simulink model "seat_sc1"  (R2020a)
settings: Solver=FixedStepDiscrete  StartTime=0.0  StopTime=30  FixedStep=1  RelTol=1e-3
settings Model: Creator=admin  LastModifiedBy=A
settings OptimizationCC: DefaultParameterBehavior=Inlined  EnhancedBackFolding=on  PassReuseOutputArgsAs=Individual arguments  OptimizeBlockOrder=speed  DifferentSizesBufferReuse=on  OptimizationCustomize=off  EfficientTunableParamExpr=on
settings DebuggingCC: ParameterTunabilityLossMsg=error
settings SFSimCC: MATLABDynamicMemAlloc=off  CustomCodeUndefinedFunction=UseInterfaceOnly
settings RTWCC: SystemTargetFile=ert.tlc  TemplateMakefile=ert_default_tmf  GenerateReport=on  IncludeHyperlinkInReport=on  LaunchReport=on  GenerateTraceInfo=on  GenerateTraceReport=on  GenerateTraceReportSl=on  GenerateTraceReportSf=on  GenerateTraceReportEml=on
settings CodeAppCC: ForceParamTrailComments=on  IgnoreCustomStorageClasses=off  OperatorAnnotations=on  SimulinkDataObjDesc=on  SFDataObjDesc=on  InsertBlockDesc=on
settings ERTTargetCC: TargetLangStandard=C99 (ISO)  GenerateSampleERTMain=on  InlinedParameterPlacement=NonHierarchical  ERTCustomFileTemplate=example_file_process.tlc

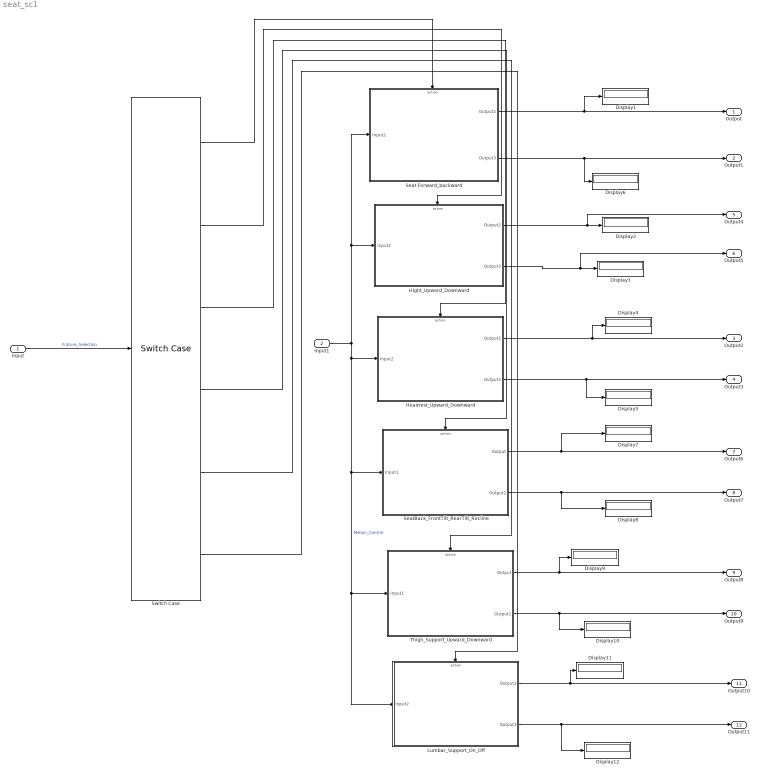
== system seat_sc1 ==
  Input : Inport
  Input1 : Inport  Port=2
  " Seat Forward_backward" : Subsystem  TreatAsAtomicUnit=on
  Display{1..12} (12 alike) : Display
  Headrest_Upward_Downward : Subsystem  TreatAsAtomicUnit=on
  Hight_Upward_Downward : Subsystem  TreatAsAtomicUnit=on
  Lumbar_Support_On_Off : Subsystem  TreatAsAtomicUnit=on
  SeatBack_FrontTilt_RearTilt_Recline : Subsystem  TreatAsAtomicUnit=on
  Switch Case : SwitchCase  CaseConditions={1 2 3 4 5 6}  ShowDefaultCase=off
  Thigh_Support_Upward_Downward : Subsystem  TreatAsAtomicUnit=on
  Output : Outport
  Output1 : Outport  Port=2
  Output2 : Outport  Port=3
  Output3 : Outport  Port=4
  Output4 : Outport  Port=5
  Output5 : Outport  Port=6
  Output6 : Outport  Port=7
  Output7 : Outport  Port=8
  Output8 : Outport  Port=9
  Output9 : Outport  Port=10
  Output10 : Outport  Port=11
  Output11 : Outport  Port=12
  wires:
  Input1/1 -> " Seat Forward_backward"/1(Input2), Hight_Upward_Downward/1(Input2), Lumbar_Support_On_Off/1(Input2), Thigh_Support_Upward_Downward/1(Input1), SeatBack_FrontTilt_RearTilt_Recline/1(Input1), Headrest_Upward_Downward/1(Input2)  "Motion_Control"
  Input/1 -> Switch Case/1  "Frature_Selection"
  Hight_Upward_Downward/1(Output2) -> Output4/1, Display2/1
  Lumbar_Support_On_Off/2(Output3) -> Output11/1, Display12/1
  Switch Case/5 -> Thigh_Support_Upward_Downward/Action
  Thigh_Support_Upward_Downward/1(Output) -> Display9/1, Output8/1
  Thigh_Support_Upward_Downward/2(Output1) -> Output9/1, Display10/1
  Headrest_Upward_Downward/1(Output2) -> Display4/1, Output2/1
  Switch Case/1 -> " Seat Forward_backward"/Action
  SeatBack_FrontTilt_RearTilt_Recline/2(Output1) -> Output7/1, Display8/1
  Switch Case/2 -> Hight_Upward_Downward/Action
  Switch Case/3 -> Headrest_Upward_Downward/Action
  Switch Case/4 -> SeatBack_FrontTilt_RearTilt_Recline/Action
  Lumbar_Support_On_Off/1(Output2) -> Output10/1, Display11/1
  SeatBack_FrontTilt_RearTilt_Recline/1(Output) -> Display7/1, Output6/1
  Switch Case/6 -> Lumbar_Support_On_Off/Action
  " Seat Forward_backward"/1(Output2) -> Display1/1, Output/1
  Headrest_Upward_Downward/2(Output3) -> Output3/1, Display5/1
  Hight_Upward_Downward/2(Output3) -> Output5/1, Display3/1
  " Seat Forward_backward"/2(Output3) -> Display6/1, Output1/1

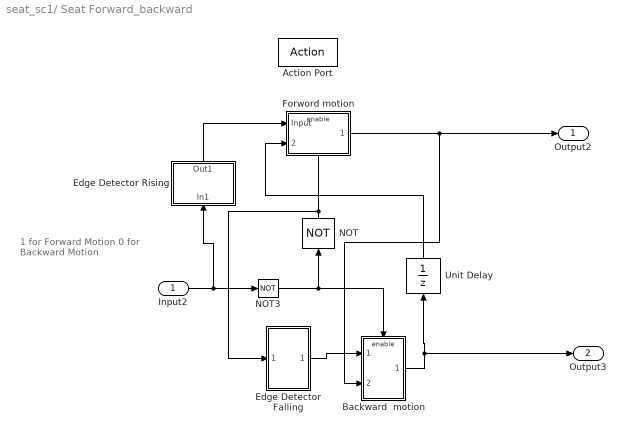
== system seat_sc1/ Seat Forward_backward ==
  note: 1 for Forward Motion
      | 0 for Backward Motion
  Input2 : Inport
  Action Port : ActionPort  ActionPortLabel=case [ 1 ]:
  " Backward  motion" : Subsystem
  Edge Detector Falling : Subsystem  TreatAsAtomicUnit=on
  Edge Detector Rising : Subsystem  TreatAsAtomicUnit=on
  Forword motion : Subsystem
  NOT : Logic  Operator=NOT  IconShape=distinctive  AllPortsSameDT=off  OutDataTypeStr=boolean
  NOT3 : Logic  Operator=NOT  IconShape=distinctive  AllPortsSameDT=off  OutDataTypeStr=boolean
  Unit Delay : UnitDelay  SampleTime=-1  HasFrameUpgradeWarning=on
  Output2 : Outport
  Output3 : Outport  Port=2
  wires:
  " Backward  motion"/1(Output) -> Output3/1, Unit Delay/1
  Edge Detector Falling/1(Out1) -> " Backward  motion"/1(Input)
  Input2/1 -> Edge Detector Rising/1(In1), NOT3/1
  Forword motion/1(Output1) -> " Backward  motion"/2(Input1), Output2/1
  NOT3/1 -> " Backward  motion"/Enable, NOT/1
  NOT/1 -> Forword motion/Enable, Edge Detector Falling/1(In1)
  Edge Detector Rising/1(Out1) -> Forword motion/1(Input)
  Unit Delay/1 -> Forword motion/2(Input1)

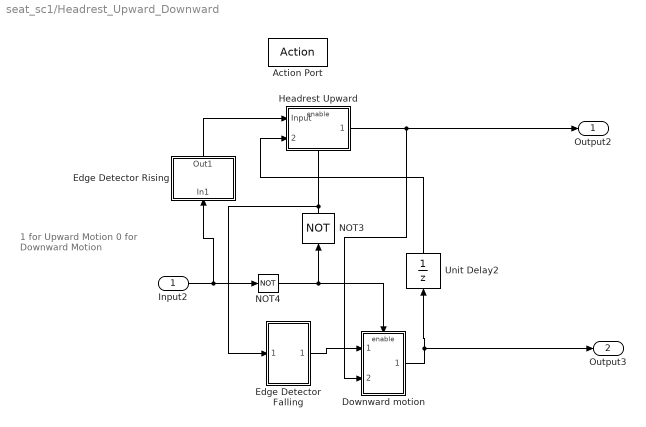
== system seat_sc1/Headrest_Upward_Downward ==
  note: 1 for Upward Motion
      | 0 for Downward Motion
  Input2 : Inport
  Action Port : ActionPort  ActionPortLabel=case [ 3 ]:
  Downward motion : Subsystem
  Edge Detector Falling : Subsystem  TreatAsAtomicUnit=on
  Edge Detector Rising : Subsystem  TreatAsAtomicUnit=on
  Headrest Upward : Subsystem
  NOT3 : Logic  Operator=NOT  IconShape=distinctive  AllPortsSameDT=off  OutDataTypeStr=boolean
  NOT4 : Logic  Operator=NOT  IconShape=distinctive  AllPortsSameDT=off  OutDataTypeStr=boolean
  Unit Delay2 : UnitDelay  SampleTime=-1  HasFrameUpgradeWarning=on
  Output2 : Outport
  Output3 : Outport  Port=2
  wires:
  Unit Delay2/1 -> Headrest Upward/2(Input1)
  Downward motion/1(Output) -> Output3/1, Unit Delay2/1
  Edge Detector Falling/1(Out1) -> Downward motion/1(Input)
  NOT4/1 -> Downward motion/Enable, NOT3/1
  Edge Detector Rising/1(Out1) -> Headrest Upward/1(Input)
  Headrest Upward/1(Output1) -> Downward motion/2(Input1), Output2/1
  NOT3/1 -> Headrest Upward/Enable, Edge Detector Falling/1(In1)
  Input2/1 -> Edge Detector Rising/1(In1), NOT4/1

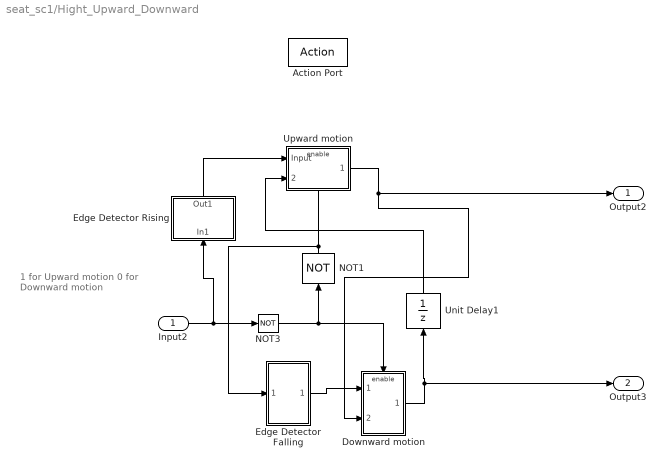
== system seat_sc1/Hight_Upward_Downward ==
  note: 1 for Upward motion
      | 0 for Downward motion
  Input2 : Inport
  Action Port : ActionPort  ActionPortLabel=case [ 2 ]:
  Downward motion : Subsystem
  Edge Detector Falling : Subsystem  TreatAsAtomicUnit=on
  Edge Detector Rising : Subsystem  TreatAsAtomicUnit=on
  NOT1 : Logic  Operator=NOT  IconShape=distinctive  AllPortsSameDT=off  OutDataTypeStr=boolean
  NOT3 : Logic  Operator=NOT  IconShape=distinctive  AllPortsSameDT=off  OutDataTypeStr=boolean
  Unit Delay1 : UnitDelay  SampleTime=-1  HasFrameUpgradeWarning=on
  Upward motion : Subsystem
  Output2 : Outport
  Output3 : Outport  Port=2
  wires:
  NOT1/1 -> Upward motion/Enable, Edge Detector Falling/1(In1)
  Edge Detector Rising/1(Out1) -> Upward motion/1(Input)
  Upward motion/1(Output1) -> Output2/1, Downward motion/2(Input1)
  NOT3/1 -> Downward motion/Enable, NOT1/1
  Edge Detector Falling/1(Out1) -> Downward motion/1(Input)
  Unit Delay1/1 -> Upward motion/2(Input1)
  Downward motion/1(Output) -> Output3/1, Unit Delay1/1
  Input2/1 -> Edge Detector Rising/1(In1), NOT3/1

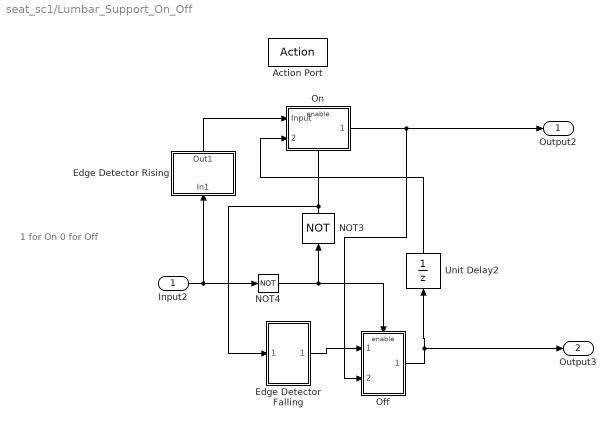
== system seat_sc1/Lumbar_Support_On_Off ==
  note: 1 for On
      | 0 for Off
  Input2 : Inport
  Action Port : ActionPort  ActionPortLabel=case [ 6 ]:
  Edge Detector Falling : Subsystem  TreatAsAtomicUnit=on
  Edge Detector Rising : Subsystem  TreatAsAtomicUnit=on
  NOT3 : Logic  Operator=NOT  IconShape=distinctive  AllPortsSameDT=off  OutDataTypeStr=boolean
  NOT4 : Logic  Operator=NOT  IconShape=distinctive  AllPortsSameDT=off  OutDataTypeStr=boolean
  Off : Subsystem
  On : Subsystem
  Unit Delay2 : UnitDelay  SampleTime=-1  HasFrameUpgradeWarning=on
  Output2 : Outport
  Output3 : Outport  Port=2
  wires:
  Input2/1 -> NOT4/1, Edge Detector Rising/1(In1)
  NOT3/1 -> Edge Detector Falling/1(In1), On/Enable
  On/1(Output1) -> Output2/1, Off/2(Input1)
  Edge Detector Rising/1(Out1) -> On/1(Input)
  NOT4/1 -> NOT3/1, Off/Enable
  Edge Detector Falling/1(Out1) -> Off/1(Input)
  Off/1(Output) -> Unit Delay2/1, Output3/1
  Unit Delay2/1 -> On/2(Input1)

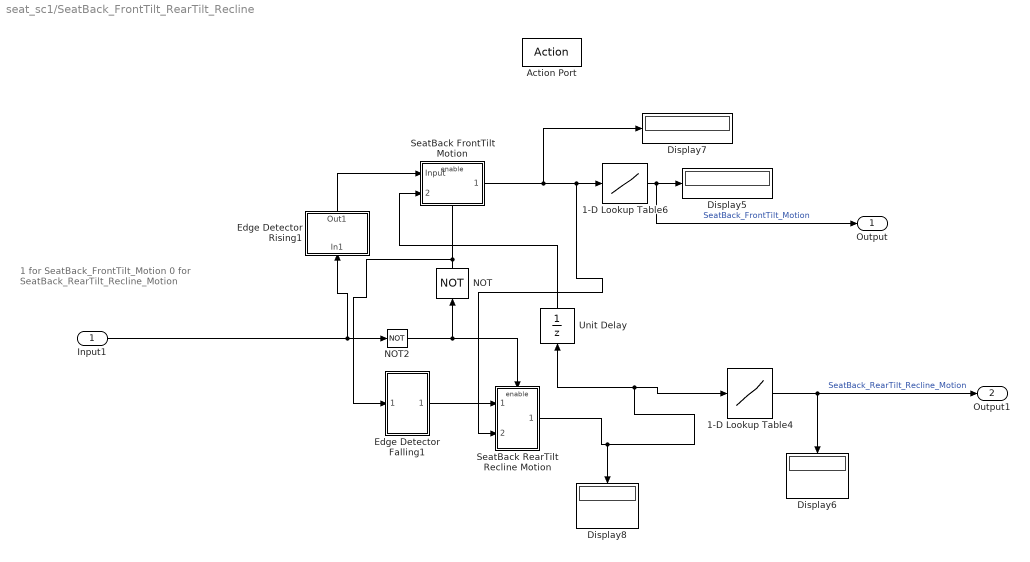
== system seat_sc1/SeatBack_FrontTilt_RearTilt_Recline ==
  note: 1 for SeatBack_FrontTilt_Motion
      | 0 for SeatBack_RearTilt_Recline_Motion
  Input1 : Inport
  Action Port : ActionPort  ActionPortLabel=case [ 4 ]:
  1-D Lookup Table4 : Lookup_n-D  NumberOfTableDimensions=1  BreakpointsForDimension1=[500 1000 1500]  Table=[70 120 170]  InternalRulePriority=Speed  RndMeth=Simplest  InputSameDT=on
  1-D Lookup Table6 : Lookup_n-D  NumberOfTableDimensions=1  BreakpointsForDimension1=[500 1000 1500]  Table=[70 120 170]  InternalRulePriority=Speed  RndMeth=Simplest  InputSameDT=on
  Display{5..8} (4 alike) : Display
  Edge Detector Falling1 : Subsystem  TreatAsAtomicUnit=on
  Edge Detector Rising1 : Subsystem  TreatAsAtomicUnit=on
  NOT : Logic  Operator=NOT  IconShape=distinctive  AllPortsSameDT=off  OutDataTypeStr=boolean
  NOT2 : Logic  Operator=NOT  IconShape=distinctive  AllPortsSameDT=off  OutDataTypeStr=boolean
  SeatBack FrontTilt Motion : Subsystem
  SeatBack RearTilt Recline Motion : Subsystem
  Unit Delay : UnitDelay  SampleTime=-1  HasFrameUpgradeWarning=on
  Output : Outport
  Output1 : Outport  Port=2
  wires:
  SeatBack FrontTilt Motion/1(Output1) -> Display7/1, 1-D Lookup Table6/1, SeatBack RearTilt Recline Motion/2(Input1)
  NOT/1 -> Edge Detector Falling1/1(In1), SeatBack FrontTilt Motion/Enable
  Input1/1 -> Edge Detector Rising1/1(In1), NOT2/1
  1-D Lookup Table6/1 -> Display5/1, Output/1  "SeatBack_FrontTilt_Motion"
  1-D Lookup Table4/1 -> Output1/1, Display6/1  "SeatBack_RearTilt_Recline_Motion"
  Unit Delay/1 -> SeatBack FrontTilt Motion/2(Input1)
  SeatBack RearTilt Recline Motion/1(Output) -> Unit Delay/1, 1-D Lookup Table4/1, Display8/1
  Edge Detector Falling1/1(Input) -> SeatBack RearTilt Recline Motion/1(Input)
  Edge Detector Rising1/1(Out1) -> SeatBack FrontTilt Motion/1(Input)
  NOT2/1 -> SeatBack RearTilt Recline Motion/Enable, NOT/1

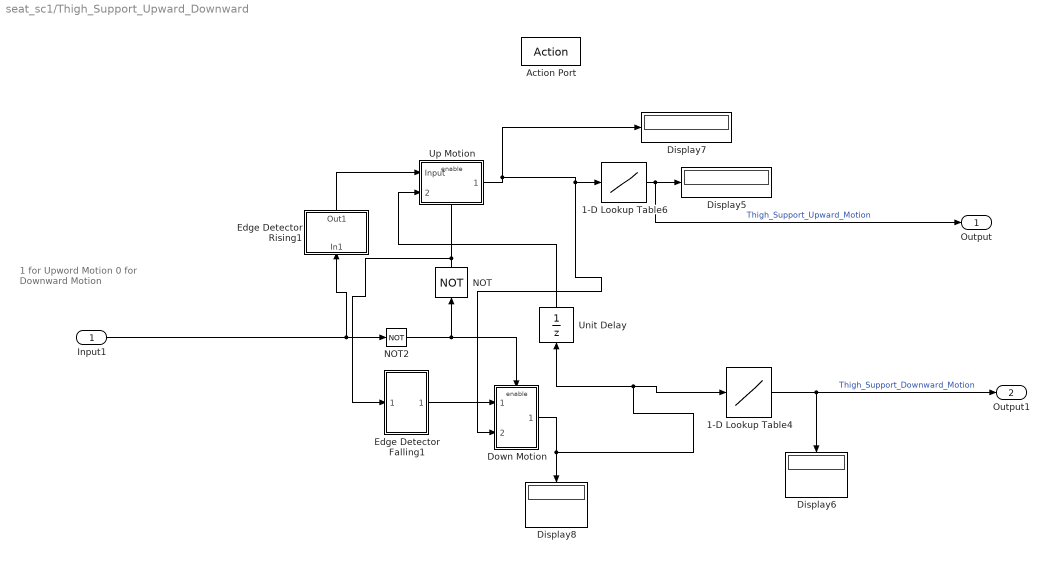
== system seat_sc1/Thigh_Support_Upward_Downward ==
  note: 1 for Upword Motion
      | 0 for Downward Motion
  Input1 : Inport
  Action Port : ActionPort  ActionPortLabel=case [ 5 ]:
  1-D Lookup Table4 : Lookup_n-D  NumberOfTableDimensions=1  BreakpointsForDimension1=[500 1000 1500]  Table=[5 10 15]  InternalRulePriority=Speed  RndMeth=Simplest  InputSameDT=on
  1-D Lookup Table6 : Lookup_n-D  NumberOfTableDimensions=1  BreakpointsForDimension1=[500 1000 1500]  Table=[5 10 15]  InternalRulePriority=Speed  RndMeth=Simplest  InputSameDT=on
  Display{5..8} (4 alike) : Display
  Down Motion : Subsystem
  Edge Detector Falling1 : Subsystem  TreatAsAtomicUnit=on
  Edge Detector Rising1 : Subsystem  TreatAsAtomicUnit=on
  NOT : Logic  Operator=NOT  IconShape=distinctive  AllPortsSameDT=off  OutDataTypeStr=boolean
  NOT2 : Logic  Operator=NOT  IconShape=distinctive  AllPortsSameDT=off  OutDataTypeStr=boolean
  Unit Delay : UnitDelay  SampleTime=-1  HasFrameUpgradeWarning=on
  Up Motion : Subsystem
  Output : Outport
  Output1 : Outport  Port=2
  wires:
  NOT2/1 -> NOT/1, Down Motion/Enable
  Edge Detector Rising1/1(Out1) -> Up Motion/1(Input)
  Edge Detector Falling1/1(Input) -> Down Motion/1(Input)
  Down Motion/1(Output) -> Display8/1, 1-D Lookup Table4/1, Unit Delay/1
  Unit Delay/1 -> Up Motion/2(Input1)
  1-D Lookup Table4/1 -> Display6/1, Output1/1  "Thigh_Support_Downward_Motion"
  1-D Lookup Table6/1 -> Output/1, Display5/1  "Thigh_Support_Upward_Motion"
  Input1/1 -> NOT2/1, Edge Detector Rising1/1(In1)
  NOT/1 -> Up Motion/Enable, Edge Detector Falling1/1(In1)
  Up Motion/1(Output1) -> Display7/1, Down Motion/2(Input1), 1-D Lookup Table6/1

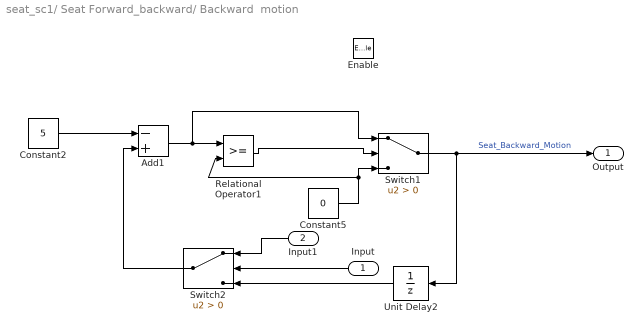
== system seat_sc1/ Seat Forward_backward/ Backward  motion ==
  Input : Inport
  Input1 : Inport  Port=2
  Enable : EnablePort
  Add1 : Sum  Inputs=-+
  Constant2 : Constant  Value=5
  Constant5 : Constant  Value=0
  Relational Operator1 : RelationalOperator  OutDataTypeStr=boolean  RndMeth=Simplest
  Switch1 : Switch  Criteria=u2 > Threshold
  Switch2 : Switch  Criteria=u2 > Threshold
  Unit Delay2 : UnitDelay  InitialCondition=200  SampleTime=-1  HasFrameUpgradeWarning=on
  Output : Outport
  wires:
  Relational Operator1/1 -> Switch1/2
  Constant2/1 -> Add1/1
  Add1/1 -> Switch1/1, Relational Operator1/1
  Constant5/1 -> Relational Operator1/2, Switch1/3
  Switch1/1 -> Unit Delay2/1, Output/1  "Seat_Backward_Motion"
  Switch2/1 -> Add1/2
  Input1/1 -> Switch2/1
  Unit Delay2/1 -> Switch2/3
  Input/1 -> Switch2/2

== system seat_sc1/ Seat Forward_backward/Edge Detector Falling ==
  In1 : Inport
  AND2 : Logic  AllPortsSameDT=off  OutDataTypeStr=boolean
  NOT1 : Logic  Operator=NOT  IconShape=distinctive  AllPortsSameDT=off  OutDataTypeStr=boolean
  Unit Delay4 : UnitDelay  InitialCondition=1  SampleTime=-1  HasFrameUpgradeWarning=on
  Out1 : Outport
  wires:
  AND2/1 -> Out1/1
  In1/1 -> NOT1/1, Unit Delay4/1
  Unit Delay4/1 -> AND2/2
  NOT1/1 -> AND2/1

== system seat_sc1/ Seat Forward_backward/Edge Detector Rising ==
  In1 : Inport
  AND2 : Logic  AllPortsSameDT=off  OutDataTypeStr=boolean
  NOT2 : Logic  Operator=NOT  IconShape=distinctive  AllPortsSameDT=off  OutDataTypeStr=boolean
  Unit Delay4 : UnitDelay  InitialCondition=1  SampleTime=-1  HasFrameUpgradeWarning=on
  Out1 : Outport
  wires:
  NOT2/1 -> AND2/2
  In1/1 -> Unit Delay4/1, AND2/1
  Unit Delay4/1 -> NOT2/1
  AND2/1 -> Out1/1

== system seat_sc1/ Seat Forward_backward/Forword motion ==
  Input : Inport
  Input1 : Inport  Port=2
  Enable : EnablePort
  Add1 : Sum
  Constant1 : Constant  Value=200
  Constant2 : Constant  Value=5
  Relational Operator1 : RelationalOperator  Operator=<=  OutDataTypeStr=boolean  RndMeth=Simplest
  Switch1 : Switch  Criteria=u2 ~= 0
  Switch2 : Switch  Criteria=u2 ~= 0
  Unit Delay2 : UnitDelay  SampleTime=-1  HasFrameUpgradeWarning=on
  Output1 : Outport
  wires:
  Constant1/1 -> Switch1/3, Relational Operator1/2
  Relational Operator1/1 -> Switch1/2
  Constant2/1 -> Add1/1
  Add1/1 -> Switch1/1, Relational Operator1/1
  Switch1/1 -> Unit Delay2/1, Output1/1  "Seat_Forward_Motion"
  Input1/1 -> Switch2/1
  Input/1 -> Switch2/2
  Unit Delay2/1 -> Switch2/3
  Switch2/1 -> Add1/2

== system seat_sc1/Headrest_Upward_Downward/Downward motion ==
  Input : Inport
  Input1 : Inport  Port=2
  Enable : EnablePort
  Add1 : Sum  Inputs=-+
  Constant2 : Constant  Value=5
  Constant5 : Constant  Value=0
  Relational Operator1 : RelationalOperator  OutDataTypeStr=boolean  RndMeth=Simplest
  Switch1 : Switch  Criteria=u2 > Threshold
  Switch2 : Switch  Criteria=u2 > Threshold
  Unit Delay2 : UnitDelay  InitialCondition=100  SampleTime=-1  HasFrameUpgradeWarning=on
  Output : Outport
  wires:
  Relational Operator1/1 -> Switch1/2
  Constant2/1 -> Add1/1
  Add1/1 -> Switch1/1, Relational Operator1/1
  Constant5/1 -> Relational Operator1/2, Switch1/3
  Switch1/1 -> Unit Delay2/1, Output/1  "Headrest_Downward_Motion"
  Switch2/1 -> Add1/2
  Input1/1 -> Switch2/1
  Unit Delay2/1 -> Switch2/3
  Input/1 -> Switch2/2

== system seat_sc1/Headrest_Upward_Downward/Edge Detector Falling ==
  In1 : Inport
  AND2 : Logic  AllPortsSameDT=off  OutDataTypeStr=boolean
  NOT1 : Logic  Operator=NOT  IconShape=distinctive  AllPortsSameDT=off  OutDataTypeStr=boolean
  Unit Delay4 : UnitDelay  InitialCondition=1  SampleTime=-1  HasFrameUpgradeWarning=on
  Out1 : Outport
  wires:
  AND2/1 -> Out1/1
  In1/1 -> NOT1/1, Unit Delay4/1
  Unit Delay4/1 -> AND2/2
  NOT1/1 -> AND2/1

== system seat_sc1/Headrest_Upward_Downward/Edge Detector Rising ==
  In1 : Inport
  AND2 : Logic  AllPortsSameDT=off  OutDataTypeStr=boolean
  NOT2 : Logic  Operator=NOT  IconShape=distinctive  AllPortsSameDT=off  OutDataTypeStr=boolean
  Unit Delay4 : UnitDelay  InitialCondition=1  SampleTime=-1  HasFrameUpgradeWarning=on
  Out1 : Outport
  wires:
  NOT2/1 -> AND2/2
  In1/1 -> Unit Delay4/1, AND2/1
  Unit Delay4/1 -> NOT2/1
  AND2/1 -> Out1/1

== system seat_sc1/Headrest_Upward_Downward/Headrest Upward ==
  Input : Inport
  Input1 : Inport  Port=2
  Enable : EnablePort
  Add1 : Sum
  Constant1 : Constant  Value=100
  Constant2 : Constant  Value=5
  Relational Operator1 : RelationalOperator  Operator=<=  OutDataTypeStr=boolean  RndMeth=Simplest
  Switch1 : Switch  Criteria=u2 ~= 0
  Switch2 : Switch  Criteria=u2 ~= 0
  Unit Delay2 : UnitDelay  SampleTime=-1  HasFrameUpgradeWarning=on
  Output1 : Outport
  wires:
  Constant1/1 -> Switch1/3, Relational Operator1/2
  Relational Operator1/1 -> Switch1/2
  Constant2/1 -> Add1/1
  Add1/1 -> Switch1/1, Relational Operator1/1
  Switch1/1 -> Unit Delay2/1, Output1/1  "Headrest_Upward_Motion"
  Input1/1 -> Switch2/1
  Input/1 -> Switch2/2
  Unit Delay2/1 -> Switch2/3
  Switch2/1 -> Add1/2

== system seat_sc1/Hight_Upward_Downward/Downward motion ==
  Input : Inport
  Input1 : Inport  Port=2
  Enable : EnablePort
  Add1 : Sum  Inputs=-+
  Constant2 : Constant  Value=5
  Constant5 : Constant  Value=0
  Relational Operator1 : RelationalOperator  OutDataTypeStr=boolean  RndMeth=Simplest
  Switch1 : Switch  Criteria=u2 > Threshold
  Switch2 : Switch  Criteria=u2 > Threshold
  Unit Delay2 : UnitDelay  InitialCondition=100  SampleTime=-1  HasFrameUpgradeWarning=on
  Output : Outport
  wires:
  Relational Operator1/1 -> Switch1/2
  Constant2/1 -> Add1/1
  Add1/1 -> Switch1/1, Relational Operator1/1
  Constant5/1 -> Relational Operator1/2, Switch1/3
  Switch1/1 -> Unit Delay2/1, Output/1  "Hight_Downward_Motion"
  Switch2/1 -> Add1/2
  Input1/1 -> Switch2/1
  Unit Delay2/1 -> Switch2/3
  Input/1 -> Switch2/2

== system seat_sc1/Hight_Upward_Downward/Edge Detector Falling ==
  In1 : Inport
  AND2 : Logic  AllPortsSameDT=off  OutDataTypeStr=boolean
  NOT1 : Logic  Operator=NOT  IconShape=distinctive  AllPortsSameDT=off  OutDataTypeStr=boolean
  Unit Delay4 : UnitDelay  InitialCondition=1  SampleTime=-1  HasFrameUpgradeWarning=on
  Out1 : Outport
  wires:
  AND2/1 -> Out1/1
  In1/1 -> NOT1/1, Unit Delay4/1
  Unit Delay4/1 -> AND2/2
  NOT1/1 -> AND2/1

== system seat_sc1/Hight_Upward_Downward/Edge Detector Rising ==
  In1 : Inport
  AND2 : Logic  AllPortsSameDT=off  OutDataTypeStr=boolean
  NOT2 : Logic  Operator=NOT  IconShape=distinctive  AllPortsSameDT=off  OutDataTypeStr=boolean
  Unit Delay4 : UnitDelay  InitialCondition=1  SampleTime=-1  HasFrameUpgradeWarning=on
  Out1 : Outport
  wires:
  NOT2/1 -> AND2/2
  In1/1 -> Unit Delay4/1, AND2/1
  Unit Delay4/1 -> NOT2/1
  AND2/1 -> Out1/1

== system seat_sc1/Hight_Upward_Downward/Upward motion ==
  Input : Inport
  Input1 : Inport  Port=2
  Enable : EnablePort
  Add1 : Sum
  Constant1 : Constant  Value=100
  Constant2 : Constant  Value=5
  Relational Operator1 : RelationalOperator  Operator=<=  OutDataTypeStr=boolean  RndMeth=Simplest
  Switch1 : Switch  Criteria=u2 ~= 0
  Switch2 : Switch  Criteria=u2 ~= 0
  Unit Delay2 : UnitDelay  SampleTime=-1  HasFrameUpgradeWarning=on
  Output1 : Outport
  wires:
  Constant1/1 -> Switch1/3, Relational Operator1/2
  Relational Operator1/1 -> Switch1/2
  Constant2/1 -> Add1/1
  Add1/1 -> Switch1/1, Relational Operator1/1
  Switch1/1 -> Unit Delay2/1, Output1/1  "Hight_Upward_Motion"
  Input1/1 -> Switch2/1
  Input/1 -> Switch2/2
  Unit Delay2/1 -> Switch2/3
  Switch2/1 -> Add1/2

== system seat_sc1/Lumbar_Support_On_Off/Edge Detector Falling ==
  In1 : Inport
  AND2 : Logic  AllPortsSameDT=off  OutDataTypeStr=boolean
  NOT1 : Logic  Operator=NOT  IconShape=distinctive  AllPortsSameDT=off  OutDataTypeStr=boolean
  Unit Delay4 : UnitDelay  InitialCondition=1  SampleTime=-1  HasFrameUpgradeWarning=on
  Out1 : Outport
  wires:
  NOT1/1 -> AND2/1
  Unit Delay4/1 -> AND2/2
  In1/1 -> Unit Delay4/1, NOT1/1
  AND2/1 -> Out1/1

== system seat_sc1/Lumbar_Support_On_Off/Edge Detector Rising ==
  In1 : Inport
  AND2 : Logic  AllPortsSameDT=off  OutDataTypeStr=boolean
  NOT2 : Logic  Operator=NOT  IconShape=distinctive  AllPortsSameDT=off  OutDataTypeStr=boolean
  Unit Delay4 : UnitDelay  InitialCondition=1  SampleTime=-1  HasFrameUpgradeWarning=on
  Out1 : Outport
  wires:
  AND2/1 -> Out1/1
  Unit Delay4/1 -> NOT2/1
  In1/1 -> AND2/1, Unit Delay4/1
  NOT2/1 -> AND2/2

== system seat_sc1/Lumbar_Support_On_Off/Off ==
  Input : Inport
  Input1 : Inport  Port=2
  Enable : EnablePort
  Add1 : Sum  Inputs=-+
  Constant2 : Constant
  Constant5 : Constant  Value=0
  Relational Operator1 : RelationalOperator  OutDataTypeStr=boolean  RndMeth=Simplest
  Switch1 : Switch  Criteria=u2 > Threshold
  Switch2 : Switch  Criteria=u2 > Threshold
  Unit Delay2 : UnitDelay  InitialCondition=3  SampleTime=-1  HasFrameUpgradeWarning=on
  Output : Outport
  wires:
  Input/1 -> Switch2/2
  Unit Delay2/1 -> Switch2/3
  Input1/1 -> Switch2/1
  Switch2/1 -> Add1/2
  Switch1/1 -> Output/1, Unit Delay2/1  "Lumbar_Support_Off"
  Constant5/1 -> Switch1/3, Relational Operator1/2
  Add1/1 -> Relational Operator1/1, Switch1/1
  Constant2/1 -> Add1/1
  Relational Operator1/1 -> Switch1/2

== system seat_sc1/Lumbar_Support_On_Off/On ==
  Input : Inport
  Input1 : Inport  Port=2
  Enable : EnablePort
  Add1 : Sum
  Constant1 : Constant  Value=3
  Constant2 : Constant
  Relational Operator1 : RelationalOperator  Operator=<=  OutDataTypeStr=boolean  RndMeth=Simplest
  Switch1 : Switch  Criteria=u2 ~= 0
  Switch2 : Switch  Criteria=u2 ~= 0
  Unit Delay2 : UnitDelay  SampleTime=-1  HasFrameUpgradeWarning=on
  Output1 : Outport
  wires:
  Switch2/1 -> Add1/2
  Unit Delay2/1 -> Switch2/3
  Input/1 -> Switch2/2
  Input1/1 -> Switch2/1
  Switch1/1 -> Output1/1, Unit Delay2/1  "Lumbar_Support_On"
  Add1/1 -> Relational Operator1/1, Switch1/1
  Constant2/1 -> Add1/1
  Relational Operator1/1 -> Switch1/2
  Constant1/1 -> Relational Operator1/2, Switch1/3

== system seat_sc1/SeatBack_FrontTilt_RearTilt_Recline/Edge Detector Falling1 ==
  In1 : Inport
  AND2 : Logic  AllPortsSameDT=off  OutDataTypeStr=boolean
  NOT1 : Logic  Operator=NOT  IconShape=distinctive  AllPortsSameDT=off  OutDataTypeStr=boolean
  Unit Delay4 : UnitDelay  InitialCondition=1  SampleTime=-1  HasFrameUpgradeWarning=on
  Input : Outport
  wires:
  AND2/1 -> Input/1
  In1/1 -> NOT1/1, Unit Delay4/1
  Unit Delay4/1 -> AND2/2
  NOT1/1 -> AND2/1

== system seat_sc1/SeatBack_FrontTilt_RearTilt_Recline/Edge Detector Rising1 ==
  In1 : Inport
  AND2 : Logic  AllPortsSameDT=off  OutDataTypeStr=boolean
  NOT2 : Logic  Operator=NOT  IconShape=distinctive  AllPortsSameDT=off  OutDataTypeStr=boolean
  Unit Delay4 : UnitDelay  InitialCondition=1  SampleTime=-1  HasFrameUpgradeWarning=on
  Out1 : Outport
  wires:
  NOT2/1 -> AND2/2
  In1/1 -> Unit Delay4/1, AND2/1
  Unit Delay4/1 -> NOT2/1
  AND2/1 -> Out1/1

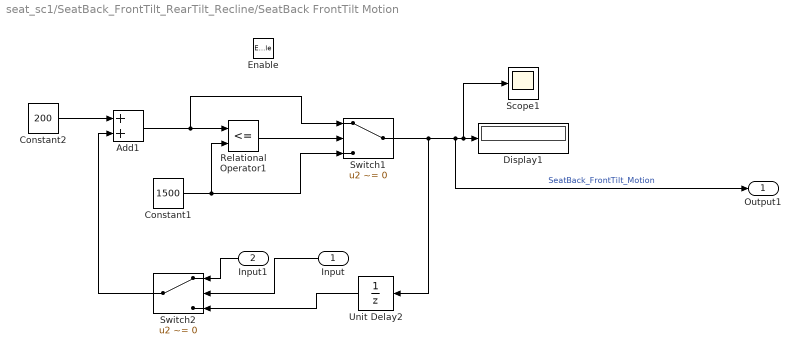
== system seat_sc1/SeatBack_FrontTilt_RearTilt_Recline/SeatBack FrontTilt Motion ==
  Input : Inport
  Input1 : Inport  Port=2
  Enable : EnablePort
  Add1 : Sum
  Constant1 : Constant  Value=1500
  Constant2 : Constant  Value=200
  Display1 : Display
  Relational Operator1 : RelationalOperator  Operator=<=  OutDataTypeStr=boolean  RndMeth=Simplest
  Scope1 : Scope
  Switch1 : Switch  Criteria=u2 ~= 0
  Switch2 : Switch  Criteria=u2 ~= 0
  Unit Delay2 : UnitDelay  SampleTime=-1  HasFrameUpgradeWarning=on
  Output1 : Outport
  wires:
  Constant1/1 -> Switch1/3, Relational Operator1/2
  Relational Operator1/1 -> Switch1/2
  Constant2/1 -> Add1/1
  Add1/1 -> Switch1/1, Relational Operator1/1
  Switch1/1 -> Unit Delay2/1, Output1/1, Scope1/1, Display1/1  "SeatBack_FrontTilt_Motion"
  Input1/1 -> Switch2/1
  Input/1 -> Switch2/2
  Unit Delay2/1 -> Switch2/3
  Switch2/1 -> Add1/2

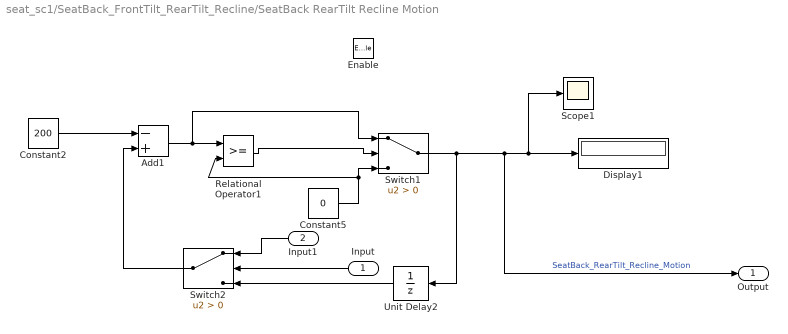
== system seat_sc1/SeatBack_FrontTilt_RearTilt_Recline/SeatBack RearTilt Recline Motion ==
  Input : Inport
  Input1 : Inport  Port=2
  Enable : EnablePort
  Add1 : Sum  Inputs=-+
  Constant2 : Constant  Value=200
  Constant5 : Constant  Value=0
  Display1 : Display
  Relational Operator1 : RelationalOperator  OutDataTypeStr=boolean  RndMeth=Simplest
  Scope1 : Scope
  Switch1 : Switch  Criteria=u2 > Threshold
  Switch2 : Switch  Criteria=u2 > Threshold
  Unit Delay2 : UnitDelay  InitialCondition=1500  SampleTime=-1  HasFrameUpgradeWarning=on
  Output : Outport
  wires:
  Relational Operator1/1 -> Switch1/2
  Constant2/1 -> Add1/1
  Add1/1 -> Switch1/1, Relational Operator1/1
  Constant5/1 -> Relational Operator1/2, Switch1/3
  Switch1/1 -> Unit Delay2/1, Output/1, Display1/1, Scope1/1  "SeatBack_RearTilt_Recline_Motion"
  Switch2/1 -> Add1/2
  Input1/1 -> Switch2/1
  Unit Delay2/1 -> Switch2/3
  Input/1 -> Switch2/2

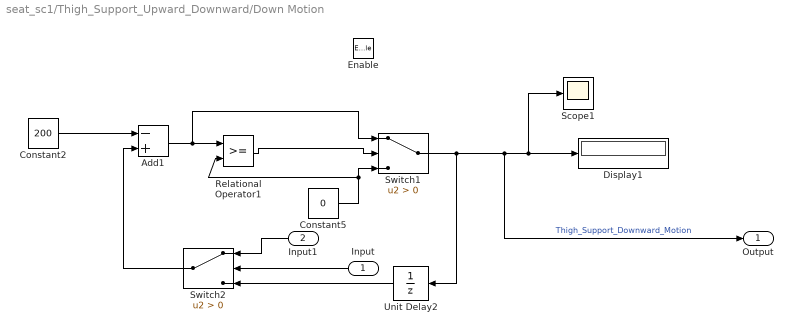
== system seat_sc1/Thigh_Support_Upward_Downward/Down Motion ==
  Input : Inport
  Input1 : Inport  Port=2
  Enable : EnablePort
  Add1 : Sum  Inputs=-+
  Constant2 : Constant  Value=200
  Constant5 : Constant  Value=0
  Display1 : Display
  Relational Operator1 : RelationalOperator  OutDataTypeStr=boolean  RndMeth=Simplest
  Scope1 : Scope
  Switch1 : Switch  Criteria=u2 > Threshold
  Switch2 : Switch  Criteria=u2 > Threshold
  Unit Delay2 : UnitDelay  InitialCondition=1500  SampleTime=-1  HasFrameUpgradeWarning=on
  Output : Outport
  wires:
  Input/1 -> Switch2/2
  Unit Delay2/1 -> Switch2/3
  Input1/1 -> Switch2/1
  Switch2/1 -> Add1/2
  Switch1/1 -> Scope1/1, Display1/1, Output/1, Unit Delay2/1  "Thigh_Support_Downward_Motion"
  Constant5/1 -> Switch1/3, Relational Operator1/2
  Add1/1 -> Relational Operator1/1, Switch1/1
  Constant2/1 -> Add1/1
  Relational Operator1/1 -> Switch1/2

== system seat_sc1/Thigh_Support_Upward_Downward/Edge Detector Falling1 ==
  In1 : Inport
  AND2 : Logic  AllPortsSameDT=off  OutDataTypeStr=boolean
  NOT1 : Logic  Operator=NOT  IconShape=distinctive  AllPortsSameDT=off  OutDataTypeStr=boolean
  Unit Delay4 : UnitDelay  InitialCondition=1  SampleTime=-1  HasFrameUpgradeWarning=on
  Input : Outport
  wires:
  NOT1/1 -> AND2/1
  Unit Delay4/1 -> AND2/2
  In1/1 -> Unit Delay4/1, NOT1/1
  AND2/1 -> Input/1

== system seat_sc1/Thigh_Support_Upward_Downward/Edge Detector Rising1 ==
  In1 : Inport
  AND2 : Logic  AllPortsSameDT=off  OutDataTypeStr=boolean
  NOT2 : Logic  Operator=NOT  IconShape=distinctive  AllPortsSameDT=off  OutDataTypeStr=boolean
  Unit Delay4 : UnitDelay  InitialCondition=1  SampleTime=-1  HasFrameUpgradeWarning=on
  Out1 : Outport
  wires:
  AND2/1 -> Out1/1
  Unit Delay4/1 -> NOT2/1
  In1/1 -> AND2/1, Unit Delay4/1
  NOT2/1 -> AND2/2

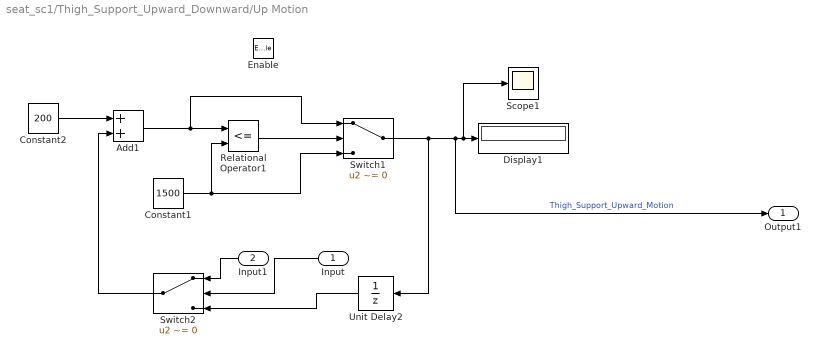
== system seat_sc1/Thigh_Support_Upward_Downward/Up Motion ==
  Input : Inport
  Input1 : Inport  Port=2
  Enable : EnablePort
  Add1 : Sum
  Constant1 : Constant  Value=1500
  Constant2 : Constant  Value=200
  Display1 : Display
  Relational Operator1 : RelationalOperator  Operator=<=  OutDataTypeStr=boolean  RndMeth=Simplest
  Scope1 : Scope
  Switch1 : Switch  Criteria=u2 ~= 0
  Switch2 : Switch  Criteria=u2 ~= 0
  Unit Delay2 : UnitDelay  SampleTime=-1  HasFrameUpgradeWarning=on
  Output1 : Outport
  wires:
  Switch2/1 -> Add1/2
  Unit Delay2/1 -> Switch2/3
  Input/1 -> Switch2/2
  Input1/1 -> Switch2/1
  Switch1/1 -> Display1/1, Scope1/1, Output1/1, Unit Delay2/1  "Thigh_Support_Upward_Motion"
  Add1/1 -> Relational Operator1/1, Switch1/1
  Constant2/1 -> Add1/1
  Relational Operator1/1 -> Switch1/2
  Constant1/1 -> Relational Operator1/2, Switch1/3
